simulink model "sample_project_closedloop_linear"  (R2023b)
settings: Solver=FixedStepAuto  StartTime=0.0  StopTime=2000  FixedStep=0.1  RelTol=1e-3
values from neighbouring files (symbols this model uses):
  A_sim = A    [sample_project.m]
  B_sim = B_u2_fail    [sample_project.m]
  C_sim = C    [sample_project.m]
  D_sim = D    [sample_project.m]
  K = place(A, B, poles)    [sample_project.m]
  u_0 = [0; 0]    [sample_project.m]
  x_0 = x_stbl - 500    [sample_project.m]
  x_stbl = [60000; 90000; 60000; 90000]    [sample_project.m]
settings Model: Creator=qingyu  LastModifiedBy=qingyu

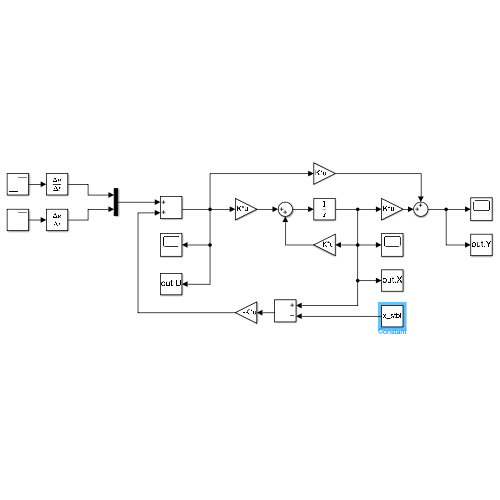
[thumbnail: Simulink's stored preview of the top-level diagram]
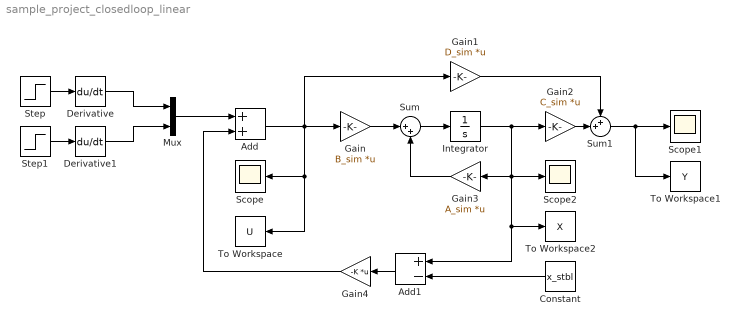
== system sample_project_closedloop_linear ==
  Add : Sum
  Add1 : Sum  Inputs=+-
  Constant : Constant  Value=x_stbl
  Derivative : Derivative
  Derivative1 : Derivative
  Gain : Gain  Gain=B_sim  Multiplication=Matrix(K*u)
  Gain1 : Gain  Gain=D_sim  Multiplication=Matrix(K*u)
  Gain2 : Gain  Gain=C_sim  Multiplication=Matrix(K*u)
  Gain3 : Gain  Gain=A_sim  Multiplication=Matrix(K*u)
  Gain4 : Gain  Gain=-K  Multiplication=Matrix(K*u)
  Integrator : Integrator  InitialCondition=x_0
  Mux : Mux  Inputs=2
  Scope : Scope
  Scope1 : Scope
  Scope2 : Scope
  Step : Step  After=u_0(1)  SampleTime=0
  Step1 : Step  After=u_0(2)  SampleTime=0
  Sum : Sum  Inputs=|++
  Sum1 : Sum  Inputs=++|
  To Workspace : ToWorkspace  VariableName=U  SampleTime=-1
  To Workspace1 : ToWorkspace  VariableName=Y  SampleTime=-1
  To Workspace2 : ToWorkspace  VariableName=X  SampleTime=-1
  wires:
  Step/1 -> Derivative/1
  Derivative/1 -> Mux/1
  Sum1/1 -> To Workspace1/1, Scope1/1
  Step1/1 -> Derivative1/1
  Derivative1/1 -> Mux/2
  Add/1 -> Gain1/1, Gain/1, To Workspace/1, Scope/1
  Gain/1 -> Sum/1
  Integrator/1 -> Gain2/1, Add1/1, To Workspace2/1, Scope2/1, Gain3/1
  Sum/1 -> Integrator/1
  Gain3/1 -> Sum/2
  Gain2/1 -> Sum1/2
  Gain1/1 -> Sum1/1
  Mux/1 -> Add/1
  Gain4/1 -> Add/2
  Add1/1 -> Gain4/1
  Constant/1 -> Add1/2
